simulink model "SS_control_sim"  (R2024b)
settings: Solver=VariableStepAuto  StartTime=0.0  StopTime=100.0  RelTol=1e-3
undefined symbols (not defined in the file): A, B, C, K, Ke, Nu, Nx
settings Model: Creator=henri  LastModifiedBy=guilherme-lazzarini
settings ConfigComp: CovBoundaryAbsTol=1.0e-5

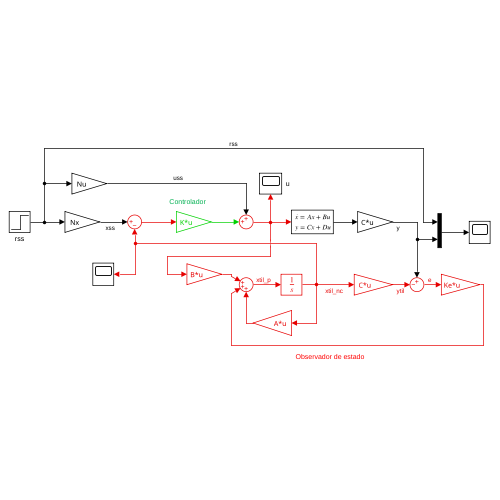
[thumbnail: Simulink's stored preview of the top-level diagram]
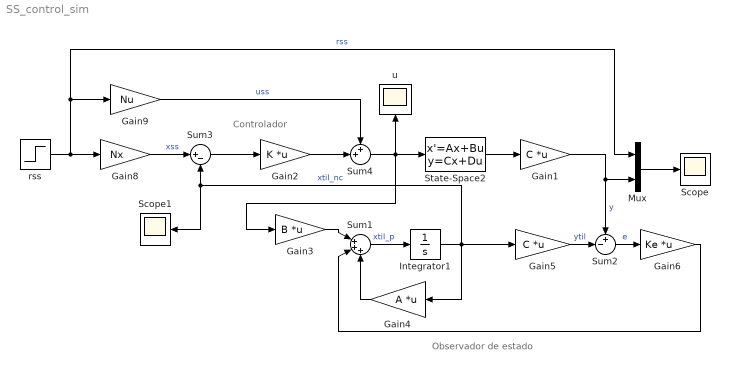
== system SS_control_sim ==
  note: Observador de estado
  note: Controlador
  Gain1 : Gain  Gain=C  Multiplication=Matrix(K*u)
  Gain2 : Gain  Gain=K  Multiplication=Matrix(K*u)
  Gain3 : Gain  Gain=B  Multiplication=Matrix(K*u)
  Gain4 : Gain  Gain=A  Multiplication=Matrix(K*u)
  Gain5 : Gain  Gain=C  Multiplication=Matrix(K*u)
  Gain6 : Gain  Gain=Ke  Multiplication=Matrix(K*u)
  Gain8 : Gain  Gain=Nx
  Gain9 : Gain  Gain=Nu
  Integrator1 : Integrator  InitialCondition=[1;1]
  Mux : Mux  Inputs=2
  Scope : Scope
  Scope1 : Scope
  State-Space2 : StateSpace  A=A  B=B  C=eye(2)  D=zeros(2,1)  InitialCondition=[0;0]
  Sum1 : Sum  Inputs=|+++
  Sum2 : Sum  Inputs=+-|
  Sum3 : Sum  Inputs=|+-
  Sum4 : Sum  Inputs=++|
  rss : Step  Time=15  After=0.8  SampleTime=0
  u : Scope
  wires:
  Sum1/1 -> Integrator1/1  "xtil_p"
  Gain9/1 -> Sum4/1  "uss"
  Sum4/1 -> Gain3/1, u/1, State-Space2/1
  Mux/1 -> Scope/1
  Gain2/1 -> Sum4/2
  Sum3/1 -> Gain2/1
  State-Space2/1 -> Gain1/1
  Gain6/1 -> Sum1/2
  Gain5/1 -> Sum2/2  "ytil"
  Gain1/1 -> Mux/2, Sum2/1  "y"
  Gain4/1 -> Sum1/3
  rss/1 -> Mux/1, Gain9/1, Gain8/1  "rss"
  Gain3/1 -> Sum1/1
  Sum2/1 -> Gain6/1  "e"
  Gain8/1 -> Sum3/1  "xss"
  Integrator1/1 -> Gain4/1, Scope1/1, Sum3/2, Gain5/1  "xtil_nc"
